simulink model "demodulate_16_bit1"  (R2021b)
settings: Solver=VariableStepAuto  StartTime=0.0  StopTime=100000/fs  RelTol=1e-3
PreLoadFcn:
  | clear all;
  | 
  | fs = 333e6
InitFcn:
  | fs = 333e6
libraries: hdlBasic x35, hdlsllib x3, dspsrcs4 x2, hdlUtilities x1, hdlDSPIP x1, simulink x1, vmcUtilities x1
settings Model: Creator=David Northcote  LastModifiedBy=clb20123
settings SolverCC: AlgebraicLoopSolver=TrustRegion
settings DataIOCC: ReturnWorkspaceOutputs=off
settings DebuggingCC: ArithmeticOperatorsInVariantConditions=warning
settings SFSimCC: SimUseLocalCustomCode=off  CustomCodeUndefinedFunction=UseInterfaceOnly
settings RTWCC: RTWUseLocalCustomCode=off  DLArmComputeVersion=20.02.1

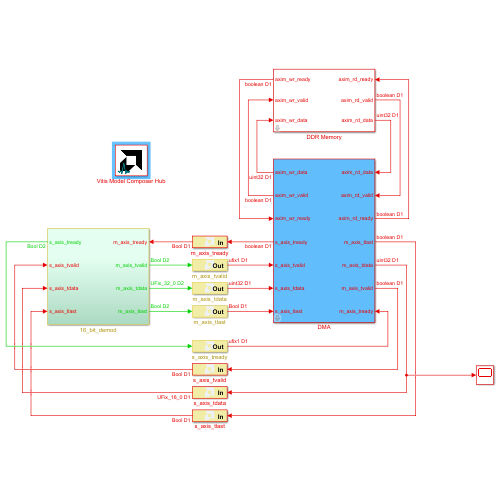
[thumbnail: Simulink's stored preview of the top-level diagram]
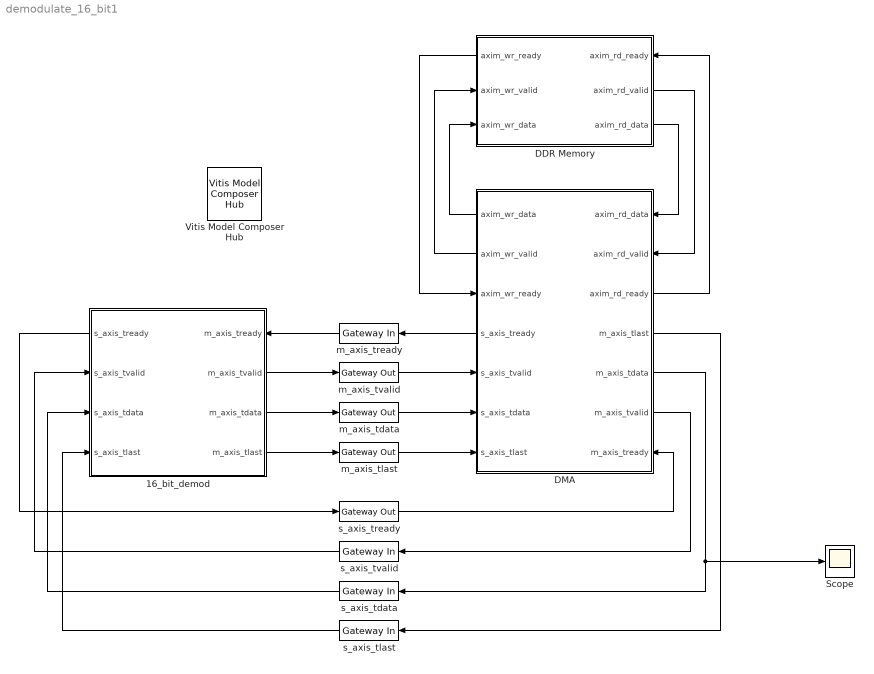
== system demodulate_16_bit1 ==
  16_bit_demod : Subsystem
      settings: PortSchema="{\"entries\":[{\"content\":{\"sides\":[{\"content\":{\"connectorIds\":[\"Out4\",\"In1\",\"In2\",\"In3\"]},\"type\":\"ConnectorPlacement.EquallySpacedRectSide\",\"uuid\":\"c102abcb-2e00-4fd7-85df-5b9b0b898bd0\"},{\"content\":{\"connectorIds\":[\"In4\",\"Out1\",\"Out2\",\"Out3\"],\"side\":\"RIGHT\"},\"type\":\"ConnectorPlacement.EquallySpacedRectSide\",\"uuid\":\"9e178eef-1e1d-41e3-971e-2eb7c6a5387e\"},{\"content\":{\"connectorIds\":[],\"side\":\"TOP\"},\"type\":\"ConnectorPlacement.EquallySpacedRectSide\",\"uuid\":\"12cf59e0-f07a-41d8-b174-5a1eb72b1624\"}]},\"type\":\"ConnectorPlacement.EquallySpacedConnector\",\"uuid\":\"cad21ed4-9065-49eb-a891-849a058d114a\"}],\"packageUris\":[\"http://schema.mathworks.com/mf0/Connector/19700101\"],\"version\":\"1.0\"}"
  DDR Memory : Subsystem  mask{bufferOut=[0 0 0 0 0 0 0 0 0 0 0], dtype=uint32, outVar='bufferIn'}
      mask prompts: bufferOut "Data to be sent:"; dtype "Data type:"; outVar "Output variable name:"
      mask init:
      | dtypeStr = get_param(gcb, 'dtype');
      | outVarStr = get_param(gcb, 'outVar');
      | set_param([gcb, '/Buffer In/To Workspace'], 'VariableName', outVar)
      settings: PortSchema="{\"entries\":[{\"content\":{\"sides\":[{\"content\":{\"connectorIds\":[\"Out3\",\"In1\",\"In2\"]},\"type\":\"ConnectorPlacement.EquallySpacedRectSide\",\"uuid\":\"10820561-fcd3-42da-ac38-14c6f993f770\"},{\"content\":{\"connectorIds\":[\"In3\",\"Out1\",\"Out2\"],\"side\":\"RIGHT\"},\"type\":\"ConnectorPlacement.EquallySpacedRectSide\",\"uuid\":\"072276f7-1cf8-495f-bb0a-1bca7e8326ea\"},{\"content\":{\"connectorIds\":[],\"side\":\"TOP\"},\"type\":\"ConnectorPlacement.EquallySpacedRectSide\",\"uuid\":\"f5b81d71-f8e7-451c-95ca-ef44dafc9f7a\"}]},\"type\":\"ConnectorPlacement.EquallySpacedConnector\",\"uuid\":\"59ea238c-ea64-4381-b9ec-a479227d5ff5\"}],\"packageUris\":[\"http://schema.mathworks.com/mf0/Connector/19700101\"],\"version\":\"1.0\"}"
      mask TypeOptions dtype: uint32 | int32
      mask DialogControl DescGroupVar Prompt: DDR Memory
      mask DialogControl DescTextVar Prompt: Block simulating a DDR memory controller.
      mask DialogControl ParameterGroupVar Prompt: MM2S
      mask DialogControl Container4 Prompt: S2MM
  DMA : Subsystem  mask{N=32}
      mask prompts: N "Length of data:"
      settings: PortSchema="{\"entries\":[{\"content\":{\"sides\":[{\"content\":{\"connectorIds\":[\"Out5\",\"Out6\",\"In1\",\"Out7\",\"In2\",\"In3\",\"In4\"]},\"type\":\"ConnectorPlacement.EquallySpacedRectSide\",\"uuid\":\"c102abcb-2e00-4fd7-85df-5b9b0b898bd0\"},{\"content\":{\"connectorIds\":[\"In5\",\"In6\",\"Out1\",\"Out2\",\"Out3\",\"Out4\",\"In7\"],\"side\":\"RIGHT\"},\"type\":\"ConnectorPlacement.EquallySpacedRectSide\",\"uuid\":\"9e178eef-1e1d-41e3-971e-2eb7c6a5387e\"},{\"content\":{\"connectorIds\":[],\"side\":\"TOP\"},\"type\":\"ConnectorPlacement.EquallySpacedRectSide\",\"uuid\":\"12cf59e0-f07a-41d8-b174-5a1eb72b1624\"},{\"content\":{\"connectorIds\":[],\"side\":\"BOTTOM\"},\"type\":\"ConnectorPlacement.EquallySpacedRectSide\",\"uuid\":\"a47cc6bb-72ec-4c9c-b625-c22428f6e2e0\"}]},\"type\":\"ConnectorPlacement.EquallySpacedConnector\",\"uuid\":\"cad21ed4-9065-49eb-a891-849a058d114a\"}],\"packageUris\":[\"http://schema.mathworks.com/mf0/Connector/19700101\"],\"version\":\"1.0\"}"
      mask DialogControl DescGroupVar Prompt: AXI DMA
      mask DialogControl DescTextVar Prompt: Block simulating an AXI DMA.
      mask DialogControl ParameterGroupVar Prompt: Main
  Scope : Scope
  Vitis Model Composer Hub : vmcUtilities/Vitis Model Composer Hub  Tag=genX  CodeGeneration=off  SubsystemName=16_bit_demod  DUTSubsystemName=16_bit_demod  CompilationType=HDLCompilation  ExportTypeV2=IP Catalog  TargetDirectory=./netlist\ip\16_bit_demod\src  exportDesign=on  analyzeDesign=off  validateDesignOnHw=off  ExportType=HDL  IpVendor=xilinx.com  IpLibrary=hls  IpVersion=1.0  IpHWLanguage=Verilog  AieCompilerOptions={}  AieSimulatorOptions={}  CreateTestbench=off  TestbenchStackSize=10  RunRtlSim=off  RunCSim=off  RunAieSim=off  AieSimTimeout=50000  RunAieSimProfiling=off  LaunchVitisAnalyzer=off  PlotOutput=off  RunX86Sim=off  X86SimTimeout=10  GenHwImage=off  GenLibadfXo=on  GenHwValidationCode=off  PlatformType=Not Specified  HwSystemType=Baremetal  HwValidationTarget=hw  ProjDevice=xczu43dr-fsve1156-2-e  ProjDevicePart=xczu43dr-fsve1156-2-e  SamplePeriod=-1  ClockFrequency=200  DataPathParallelism=1  xilinxfamily=zynquplusRFSOC  part=xczu43dr  speed=-2-e  package=fsve1156  directory=./netlist\ip\16_bit_demod\src  testbench=off  incr_netlist=off  synthesis_tool=Vivado  clock_wrapper=Clock Enables  dbl_ovrd=According to Block Masks  dcm_input_clock_period=10  sysclk_period=3.003  simulink_period=1/fs  eval_field=0  IPInfoJsonString="{\"HDLSubsystem\":{\"SubsystemName\":\"16_bit_demod\",\"IPName\":\"DUT\",\"IPLibrary\":\"VMC\",\"IPVendor\":\"User Company\",\"IPVersion\":\"1.0\",\"TargetDirectory\":\"./netlist\",\"SubsystemDir\":\"./netlist\\\\ip\\\\16_bit_demod\"},\"SubsystemTag\":\"HDLNode\"}"  LogFileName=''  NThreads=4
  m_axis_tdata : hdlBasic/Gateway Out  inherit_from_input=on  hdl_port=on  rows=1  columns=1  UseAsDAC=off  DACChannel='1'  interface=None  automatic_assignment=on  address_offset=hex2dec('00')  intf_name=''  intf_description=''  timing_constraint=None  locs_specified=off  LOCs={}  io_standard={}  XmcBlockStatus=1  maskContainerNames=group4  block_type=gatewayout  block_config=sysgen:gateway_out_config  block_width_w=590  block_height_w=620  block_width=620  block_height=750
  m_axis_tlast : hdlBasic/Gateway Out  inherit_from_input=on  hdl_port=on  rows=1  columns=1  UseAsDAC=off  DACChannel='1'  interface=None  automatic_assignment=on  address_offset=hex2dec('00')  intf_name=''  intf_description=''  timing_constraint=None  locs_specified=off  LOCs={}  io_standard={}  XmcBlockStatus=1  maskContainerNames=group4  block_type=gatewayout  block_config=sysgen:gateway_out_config  block_width_w=590  block_height_w=620  block_width=620  block_height=750
  m_axis_tready : hdlBasic/Gateway In  gui_display_data_type=Boolean  arith_type=Boolean  n_bits=16  bin_pt=14  preci_type=Single  exp_width=8  frac_width=24  rows=1  columns=1  quantization="Round  (unbiased: +/- Inf)"  overflow=Saturate  period=1/fs  UseAsADC=off  ADCChannel='1'  interface=None  automatic_assignment=on  address_offset=hex2dec('00')  intf_name=''  intf_description=''  default_value=0  timing_constraint=None  locs_specified=off  LOCs={}  io_standard={}  inherit_from_input=off  hdl_port=on  XmcBlockStatus=1  maskContainerNames=group4  block_type=gatewayin  block_config=sysgen:gateway_in_config  block_width_w=590  block_height_w=620  block_width=640  block_height=850
  m_axis_tvalid : hdlBasic/Gateway Out  inherit_from_input=on  hdl_port=on  rows=1  columns=1  UseAsDAC=off  DACChannel='1'  interface=None  automatic_assignment=on  address_offset=hex2dec('00')  intf_name=''  intf_description=''  timing_constraint=None  locs_specified=off  LOCs={}  io_standard={}  XmcBlockStatus=1  maskContainerNames=group4  block_type=gatewayout  block_config=sysgen:gateway_out_config  block_width_w=590  block_height_w=620  block_width=620  block_height=750
  s_axis_tdata : hdlBasic/Gateway In  gui_display_data_type=Fixed-point  arith_type=Unsigned  n_bits=16  bin_pt=0  preci_type=Single  exp_width=8  frac_width=24  rows=1  columns=1  quantization="Round  (unbiased: +/- Inf)"  overflow=Saturate  period=1/fs  UseAsADC=off  ADCChannel='1'  interface=None  automatic_assignment=on  address_offset=hex2dec('00')  intf_name=''  intf_description=''  default_value=0  timing_constraint=None  locs_specified=off  LOCs={}  io_standard={}  inherit_from_input=off  hdl_port=on  XmcBlockStatus=1  maskContainerNames=group4  block_type=gatewayin  block_config=sysgen:gateway_in_config  block_width_w=590  block_height_w=620  block_width=640  block_height=850
  s_axis_tlast : hdlBasic/Gateway In  gui_display_data_type=Boolean  arith_type=Boolean  n_bits=16  bin_pt=14  preci_type=Single  exp_width=8  frac_width=24  rows=1  columns=1  quantization="Round  (unbiased: +/- Inf)"  overflow=Saturate  period=1/fs  UseAsADC=off  ADCChannel='1'  interface=None  automatic_assignment=on  address_offset=hex2dec('00')  intf_name=''  intf_description=''  default_value=0  timing_constraint=None  locs_specified=off  LOCs={}  io_standard={}  inherit_from_input=off  hdl_port=on  XmcBlockStatus=1  maskContainerNames=group4  block_type=gatewayin  block_config=sysgen:gateway_in_config  block_width_w=590  block_height_w=620  block_width=640  block_height=850
  s_axis_tready : hdlBasic/Gateway Out  inherit_from_input=on  hdl_port=on  rows=1  columns=1  UseAsDAC=off  DACChannel='1'  interface=None  automatic_assignment=on  address_offset=hex2dec('00')  intf_name=''  intf_description=''  timing_constraint=None  locs_specified=off  LOCs={}  io_standard={}  XmcBlockStatus=1  maskContainerNames=group4  block_type=gatewayout  block_config=sysgen:gateway_out_config  block_width_w=590  block_height_w=620  block_width=620  block_height=750
  s_axis_tvalid : hdlBasic/Gateway In  gui_display_data_type=Boolean  arith_type=Boolean  n_bits=16  bin_pt=14  preci_type=Single  exp_width=8  frac_width=24  rows=1  columns=1  quantization="Round  (unbiased: +/- Inf)"  overflow=Saturate  period=1/fs  UseAsADC=off  ADCChannel='1'  interface=None  automatic_assignment=on  address_offset=hex2dec('00')  intf_name=''  intf_description=''  default_value=0  timing_constraint=None  locs_specified=off  LOCs={}  io_standard={}  inherit_from_input=off  hdl_port=on  XmcBlockStatus=1  maskContainerNames=group4  block_type=gatewayin  block_config=sysgen:gateway_in_config  block_width_w=590  block_height_w=620  block_width=640  block_height=850
  wires:
  s_axis_tvalid/1 -> 16_bit_demod/1(s_axis_tvalid)
  s_axis_tdata/1 -> 16_bit_demod/2(s_axis_tdata)
  s_axis_tlast/1 -> 16_bit_demod/3(s_axis_tlast)
  m_axis_tready/1 -> 16_bit_demod/4(m_axis_tready)
  16_bit_demod/4(s_axis_tready) -> s_axis_tready/1
  16_bit_demod/2(m_axis_tdata) -> m_axis_tdata/1
  16_bit_demod/1(m_axis_tvalid) -> m_axis_tvalid/1
  16_bit_demod/3(m_axis_tlast) -> m_axis_tlast/1
  s_axis_tready/1 -> DMA/7(m_axis_tready)
  DMA/4(m_axis_tvalid) -> s_axis_tvalid/1
  DMA/3(m_axis_tdata) -> Scope/1, s_axis_tdata/1
  DMA/2(m_axis_tlast) -> s_axis_tlast/1
  DMA/7(s_axis_tready) -> m_axis_tready/1
  m_axis_tvalid/1 -> DMA/2(s_axis_tvalid)
  m_axis_tdata/1 -> DMA/3(s_axis_tdata)
  m_axis_tlast/1 -> DMA/4(s_axis_tlast)
  DMA/1(axim_rd_ready) -> DDR Memory/3(axim_rd_ready)
  DDR Memory/1(axim_rd_valid) -> DMA/6(axim_rd_valid)
  DDR Memory/2(axim_rd_data) -> DMA/5(axim_rd_data)
  DDR Memory/3(axim_wr_ready) -> DMA/1(axim_wr_ready)
  DMA/6(axim_wr_valid) -> DDR Memory/1(axim_wr_valid)
  DMA/5(axim_wr_data) -> DDR Memory/2(axim_wr_data)

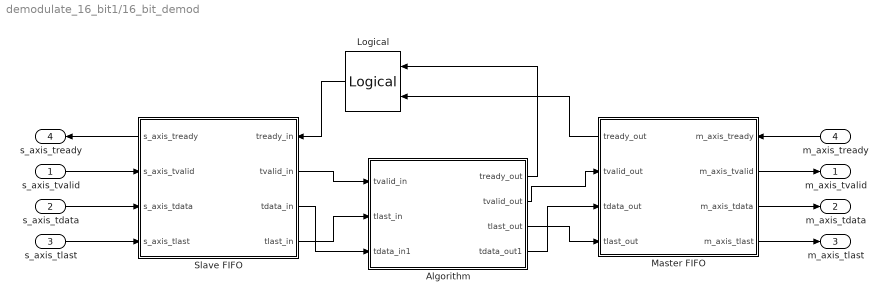
== system demodulate_16_bit1/16_bit_demod ==
  s_axis_tvalid : Inport
  s_axis_tdata : Inport  Port=2
  s_axis_tlast : Inport  Port=3
  m_axis_tready : Inport  Port=4
  Algorithm : Subsystem
  Logical : hdlBasic/Logical  logical_function=AND  inputs=2  en=off  latency=0  precision=Full  arith_type=Unsigned  n_bits=16  bin_pt=0  align_bp=on  overflow=[]  quantization=[]  XmcBlockStatus=1  maskContainerNames=tabcontainer1  block_type=logical  block_config=sysgen:Logical_config
  Master FIFO : Subsystem
      settings: PortSchema="{\"entries\":[{\"content\":{\"sides\":[{\"content\":{\"connectorIds\":[\"Out4\",\"In1\",\"In2\",\"In3\"]},\"type\":\"ConnectorPlacement.EquallySpacedRectSide\",\"uuid\":\"10820561-fcd3-42da-ac38-14c6f993f770\"},{\"content\":{\"connectorIds\":[\"In4\",\"Out1\",\"Out2\",\"Out3\"],\"side\":\"RIGHT\"},\"type\":\"ConnectorPlacement.EquallySpacedRectSide\",\"uuid\":\"072276f7-1cf8-495f-bb0a-1bca7e8326ea\"},{\"content\":{\"connectorIds\":[],\"side\":\"TOP\"},\"type\":\"ConnectorPlacement.EquallySpacedRectSide\",\"uuid\":\"f5b81d71-f8e7-451c-95ca-ef44dafc9f7a\"}]},\"type\":\"ConnectorPlacement.EquallySpacedConnector\",\"uuid\":\"59ea238c-ea64-4381-b9ec-a479227d5ff5\"}],\"packageUris\":[\"http://schema.mathworks.com/mf0/Connector/19700101\"],\"version\":\"1.0\"}"
  Slave FIFO : Subsystem
      settings: PortSchema="{\"entries\":[{\"content\":{\"sides\":[{\"content\":{\"connectorIds\":[\"Out4\",\"In1\",\"In2\",\"In3\"]},\"type\":\"ConnectorPlacement.EquallySpacedRectSide\",\"uuid\":\"10820561-fcd3-42da-ac38-14c6f993f770\"},{\"content\":{\"connectorIds\":[\"In4\",\"Out1\",\"Out2\",\"Out3\"],\"side\":\"RIGHT\"},\"type\":\"ConnectorPlacement.EquallySpacedRectSide\",\"uuid\":\"072276f7-1cf8-495f-bb0a-1bca7e8326ea\"},{\"content\":{\"connectorIds\":[],\"side\":\"TOP\"},\"type\":\"ConnectorPlacement.EquallySpacedRectSide\",\"uuid\":\"f5b81d71-f8e7-451c-95ca-ef44dafc9f7a\"}]},\"type\":\"ConnectorPlacement.EquallySpacedConnector\",\"uuid\":\"59ea238c-ea64-4381-b9ec-a479227d5ff5\"}],\"packageUris\":[\"http://schema.mathworks.com/mf0/Connector/19700101\"],\"version\":\"1.0\"}"
  m_axis_tvalid : Outport  VectorParamsAs1DForOutWhenUnconnected=off
  m_axis_tdata : Outport  Port=2  VectorParamsAs1DForOutWhenUnconnected=off
  m_axis_tlast : Outport  Port=3  VectorParamsAs1DForOutWhenUnconnected=off
  s_axis_tready : Outport  Port=4  VectorParamsAs1DForOutWhenUnconnected=off
  wires:
  Master FIFO/1(m_axis_tvalid) -> m_axis_tvalid/1
  Master FIFO/2(m_axis_tdata) -> m_axis_tdata/1
  Master FIFO/3(m_axis_tlast) -> m_axis_tlast/1
  Algorithm/2(tvalid_out) -> Master FIFO/1(tvalid_out)
  Algorithm/4(tdata_out1) -> Master FIFO/2(tdata_out)
  Algorithm/3(tlast_out) -> Master FIFO/3(tlast_out)
  s_axis_tvalid/1 -> Slave FIFO/1(s_axis_tvalid)
  s_axis_tdata/1 -> Slave FIFO/2(s_axis_tdata)
  s_axis_tlast/1 -> Slave FIFO/3(s_axis_tlast)
  Slave FIFO/1(tvalid_in) -> Algorithm/1(tvalid_in)
  Slave FIFO/3(tlast_in) -> Algorithm/2(tlast_in)
  Slave FIFO/4(s_axis_tready) -> s_axis_tready/1
  m_axis_tready/1 -> Master FIFO/4(m_axis_tready)
  Algorithm/1(tready_out) -> Logical/1
  Master FIFO/4(tready_out) -> Logical/2
  Logical/1 -> Slave FIFO/4(tready_in)
  Slave FIFO/2(tdata_in) -> Algorithm/3(tdata_in1)

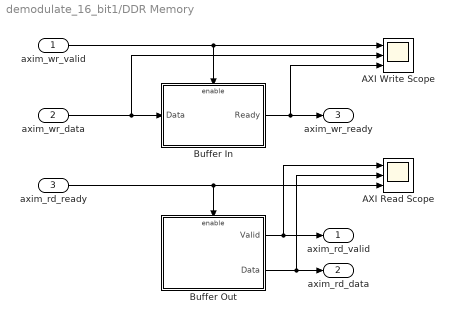
== system demodulate_16_bit1/DDR Memory ==
  axim_wr_valid : Inport
  axim_wr_data : Inport  Port=2
  axim_rd_ready : Inport  Port=3
  AXI Read Scope : Scope  NumInputPorts=3
  AXI Write Scope : Scope  NumInputPorts=3
  Buffer In : Subsystem
  Buffer Out : Subsystem
  axim_rd_valid : Outport
  axim_rd_data : Outport  Port=2
  axim_wr_ready : Outport  Port=3
  wires:
  Buffer Out/1(Valid) -> AXI Read Scope/1, axim_rd_valid/1
  Buffer Out/2(Data) -> AXI Read Scope/2, axim_rd_data/1
  axim_rd_ready/1 -> Buffer Out/Enable, AXI Read Scope/3
  axim_wr_data/1 -> AXI Write Scope/2, Buffer In/1(Data)
  Buffer In/1(Ready) -> AXI Write Scope/3, axim_wr_ready/1
  axim_wr_valid/1 -> Buffer In/Enable, AXI Write Scope/1

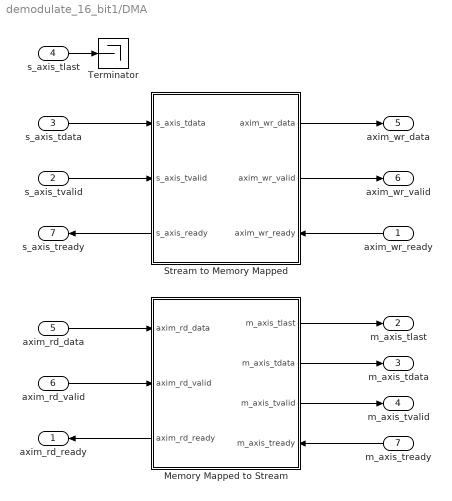
== system demodulate_16_bit1/DMA ==
  axim_wr_ready : Inport
  s_axis_tvalid : Inport  Port=2
  s_axis_tdata : Inport  Port=3
  s_axis_tlast : Inport  Port=4
  axim_rd_data : Inport  Port=5
  axim_rd_valid : Inport  Port=6
  m_axis_tready : Inport  Port=7
  Memory Mapped to Stream : Subsystem
      settings: PortSchema="{\"entries\":[{\"content\":{\"sides\":[{\"content\":{\"connectorIds\":[\"In1\",\"In2\",\"Out4\"]},\"type\":\"ConnectorPlacement.EquallySpacedRectSide\",\"uuid\":\"10820561-fcd3-42da-ac38-14c6f993f770\"},{\"content\":{\"connectorIds\":[\"Out1\",\"Out2\",\"Out3\",\"In3\"],\"side\":\"RIGHT\"},\"type\":\"ConnectorPlacement.EquallySpacedRectSide\",\"uuid\":\"072276f7-1cf8-495f-bb0a-1bca7e8326ea\"},{\"content\":{\"connectorIds\":[],\"side\":\"TOP\"},\"type\":\"ConnectorPlacement.EquallySpacedRectSide\",\"uuid\":\"f5b81d71-f8e7-451c-95ca-ef44dafc9f7a\"}]},\"type\":\"ConnectorPlacement.EquallySpacedConnector\",\"uuid\":\"59ea238c-ea64-4381-b9ec-a479227d5ff5\"}],\"packageUris\":[\"http://schema.mathworks.com/mf0/Connector/19700101\"],\"version\":\"1.0\"}"
  Stream to Memory Mapped : Subsystem
      settings: PortSchema="{\"entries\":[{\"content\":{\"sides\":[{\"content\":{\"connectorIds\":[\"In1\",\"In2\",\"Out3\"]},\"type\":\"ConnectorPlacement.EquallySpacedRectSide\",\"uuid\":\"10820561-fcd3-42da-ac38-14c6f993f770\"},{\"content\":{\"connectorIds\":[\"Out1\",\"Out2\",\"In3\"],\"side\":\"RIGHT\"},\"type\":\"ConnectorPlacement.EquallySpacedRectSide\",\"uuid\":\"072276f7-1cf8-495f-bb0a-1bca7e8326ea\"},{\"content\":{\"connectorIds\":[],\"side\":\"TOP\"},\"type\":\"ConnectorPlacement.EquallySpacedRectSide\",\"uuid\":\"f5b81d71-f8e7-451c-95ca-ef44dafc9f7a\"}]},\"type\":\"ConnectorPlacement.EquallySpacedConnector\",\"uuid\":\"59ea238c-ea64-4381-b9ec-a479227d5ff5\"}],\"packageUris\":[\"http://schema.mathworks.com/mf0/Connector/19700101\"],\"version\":\"1.0\"}"
  Terminator : Terminator
  axim_rd_ready : Outport
  m_axis_tlast : Outport  Port=2  VectorParamsAs1DForOutWhenUnconnected=off
  m_axis_tdata : Outport  Port=3  VectorParamsAs1DForOutWhenUnconnected=off
  m_axis_tvalid : Outport  Port=4  VectorParamsAs1DForOutWhenUnconnected=off
  axim_wr_data : Outport  Port=5
  axim_wr_valid : Outport  Port=6
  s_axis_tready : Outport  Port=7  VectorParamsAs1DForOutWhenUnconnected=off
  wires:
  m_axis_tready/1 -> Memory Mapped to Stream/3(m_axis_tready)
  Memory Mapped to Stream/1(m_axis_tlast) -> m_axis_tlast/1
  Memory Mapped to Stream/2(m_axis_tdata) -> m_axis_tdata/1
  Memory Mapped to Stream/3(m_axis_tvalid) -> m_axis_tvalid/1
  s_axis_tvalid/1 -> Stream to Memory Mapped/2(s_axis_tvalid)
  s_axis_tdata/1 -> Stream to Memory Mapped/1(s_axis_tdata)
  Stream to Memory Mapped/3(s_axis_ready) -> s_axis_tready/1
  s_axis_tlast/1 -> Terminator/1
  Stream to Memory Mapped/1(axim_wr_data) -> axim_wr_data/1
  Stream to Memory Mapped/2(axim_wr_valid) -> axim_wr_valid/1
  axim_wr_ready/1 -> Stream to Memory Mapped/3(axim_wr_ready)
  Memory Mapped to Stream/4(axim_rd_ready) -> axim_rd_ready/1
  axim_rd_data/1 -> Memory Mapped to Stream/1(axim_rd_data)
  axim_rd_valid/1 -> Memory Mapped to Stream/2(axim_rd_valid)

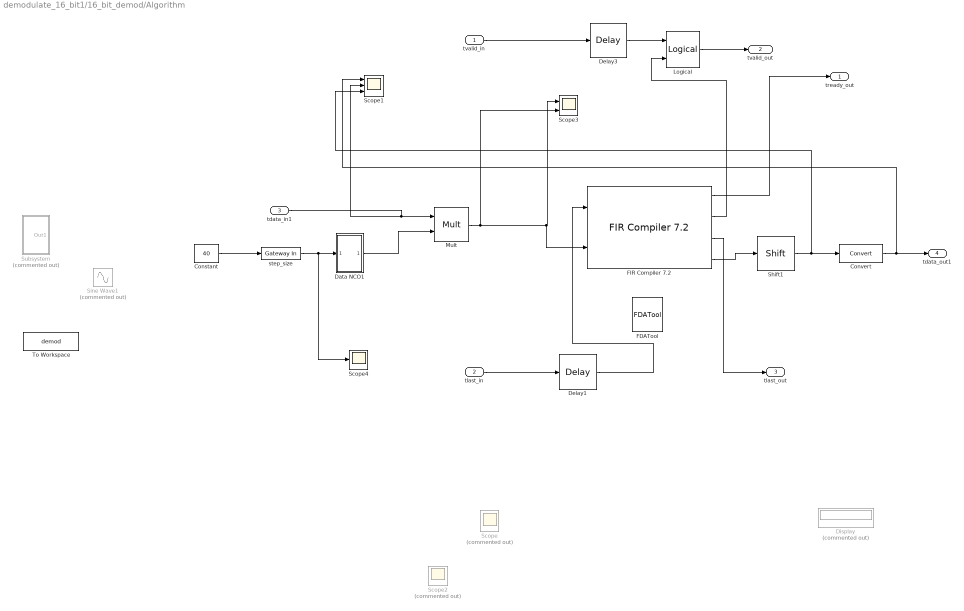
== system demodulate_16_bit1/16_bit_demod/Algorithm ==
  tvalid_in : Inport
  tlast_in : Inport  Port=2
  tdata_in1 : Inport  Port=3
  Constant : Constant  Value=40
  Convert : hdlBasic/Convert  gui_display_data_type=Fixed-point  arith_type=Unsigned  n_bits=32  bin_pt=0  float_type=Single  exp_bits=8  fraction_bits=24  quantization=Truncate  overflow=Wrap  en=off  latency=1  pipeline=off  XmcBlockStatus=1  maskContainerNames=group2  block_type=convert  block_config=sysgen:Convert_config  block_width=595  block_height=885
  Data NCO1 : Subsystem
  Delay1 : hdlBasic/Delay  rst=off  en=off  latency=9  reg_retiming=off  XmcBlockStatus=1  maskContainerNames=group1  block_type=delay  block_config=sysgen:Delay_config
  Delay3 : hdlBasic/Delay  rst=off  en=off  latency=9  reg_retiming=off  XmcBlockStatus=1  maskContainerNames=group1  block_type=delay  block_config=sysgen:Delay_config
  Display : Display  Commented=on
  FDATool : hdlUtilities/FDATool  block_type=fdatool
      settings: infoedit=FDATool
  FIR Compiler 7.2 : hdlDSPIP/FIR Compiler 7.2   coefficientvector=coeff  coefficient_sets=1  coefficient_reload=off  filter_type=Single_Rate  rate_change_type=Integer  interpolation_rate=1  decimation_rate=1  zero_pack_factor=1  channel_sequence=Basic  number_channels=1  pattern_list='P4-0,P4-1,P4-2,P4-3,P4-4'  number_paths=1  ratespecification=Maximum_Possible  sampleperiod=1  hardwareoversamplingrate=1  coefficient_sign=Signed  quantization=Normalize_to_Centre_Coefficient  coefficient_width=16  bestprecision=off  coefficient_fractional_bits=0  coefficient_structure=Inferred  output_rounding_mode=Full_Precision  output_width=31  filter_architecture=Systolic_Multiply_Accumulate  optimization_goal=Area  optimization_list='None'  data_buffer_type=Automatic  coefficient_buffer_type=Automatic  input_buffer_type=Automatic  output_buffer_type=Automatic  preference_for_other_storage=Automatic  multi_column_support=Automatic  columnconfig='101'  inter_column_pipe_length=4  data_has_tlast=Packet_Framing  m_data_has_tready=off  s_data_has_fifo=off  s_data_has_tuser=Not_Required  m_data_has_tuser=Not_Required  s_config_sync_mode=On_Vector  s_config_method=Single  num_reload_slots=1  has_aclken=off  has_aresetn=off  reset_data_vector=on  trim_axipin_name=on  simulation_type=hybrid_sim  simulation_model=sysgen:xfirv7_2_cmodel  data_path_portlist={ 's_axis_data_tdata', 'm_axis_data_tdata' }  passband_min=0.0  passband_max=0.5  stopband_min=0.5  stopband_max=1.0  filter_selection=1  gui_behaviour='Sysgen_GUI'  data_sign=Signed  data_width=16  data_fractional_bits=0  data_tuser_width=1  wrapper_available=true  ip_wrap_arbitrary_binary_point=true  ip_name=FIR Compiler  ip_version=7.2  dsptool_ready=true  ipcore_usecache=true  ipcore_useipmodelcache=true  port_translation_map={ 'aclken' => 'en', 'aresetn' => 'rst' }  run_core_at_system_period=true  ipcore_xco_need_fpga_part=true  ipcore_fpga_part=[]  XmcBlockStatus=1  maskContainerNames=tabcontainer1  block_type=fir_compiler_v7_2  block_config=sysgen:rodinimport_config  block_width=820  block_height=600
  Logical : hdlBasic/Logical  logical_function=AND  inputs=2  en=off  latency=0  precision=Full  arith_type=Unsigned  n_bits=16  bin_pt=0  align_bp=on  overflow=[]  quantization=[]  XmcBlockStatus=1  maskContainerNames=tabcontainer1  block_type=logical  block_config=sysgen:Logical_config
  Mult : hdlBasic/Mult  precision=Full  arith_type="Signed  (2's comp)"  n_bits=16  bin_pt=8  quantization=Truncate  overflow=Wrap  en=off  latency=3  use_behavioral_HDL=off  opt=Speed  use_embedded=on  optimum_pipeline=off  pipeline=on  use_rpm=on  placement_style=Triangular  XmcBlockStatus=1  maskContainerNames=group1  block_type=mult  block_config=sysgen:Mult_config  block_width=598  block_height=876
  Scope : Scope  Commented=on
  Scope1 : Scope  NumInputPorts=3
  Scope2 : Scope  Commented=on
  Scope3 : Scope  NumInputPorts=2
  Scope4 : Scope
  Shift1 : hdlBasic/Shift  shift_dir=Left  shift_bits=15  en=off  latency=1  precision=User Defined  arith_type="Signed  (2's comp)"  n_bits=47  bin_pt=0  quantization="Round  (unbiased: +/- Inf)"  overflow=Saturate  XmcBlockStatus=1  maskContainerNames=group2  block_type=shift  block_config=sysgen:Shift_config
  Sine Wave1 : Sin  Commented=on  Frequency=31415926.534298  SampleTime=0
  Subsystem : Subsystem  Commented=on
  To Workspace : ToWorkspace  VariableName=demod  SaveFormat=Timeseries  SampleTime=-1
  step_size : hdlBasic/Gateway In  gui_display_data_type=Fixed-point  arith_type=Signed (2's comp)  n_bits=16  bin_pt=8  preci_type=Single  exp_width=8  frac_width=24  rows=1  columns=1  quantization="Round  (unbiased: +/- Inf)"  overflow=Saturate  period=1/fs  UseAsADC=off  ADCChannel='1'  interface=None  automatic_assignment=on  address_offset=hex2dec('00')  intf_name=''  intf_description=''  default_value=0  timing_constraint=None  locs_specified=off  LOCs={}  io_standard={}  inherit_from_input=off  hdl_port=on  XmcBlockStatus=1  maskContainerNames=group4  block_type=gatewayin  block_config=sysgen:gateway_in_config  block_width_w=590  block_height_w=620  block_width=640  block_height=850
  tready_out : Outport
  tvalid_out : Outport  Port=2  VectorParamsAs1DForOutWhenUnconnected=off
  tlast_out : Outport  Port=3  VectorParamsAs1DForOutWhenUnconnected=off
  tdata_out1 : Outport  Port=4  VectorParamsAs1DForOutWhenUnconnected=off
  wires:
  tvalid_in/1 -> Delay3/1
  Delay1/1 -> FIR Compiler 7.2/1
  tlast_in/1 -> Delay1/1
  Delay3/1 -> Logical/1
  Logical/1 -> tvalid_out/1
  Shift1/1 -> Scope1/3, Convert/1
  step_size/1 -> Data NCO1/1(In1), Scope4/1
  Mult/1 -> FIR Compiler 7.2/2, Scope3/1, Scope3/2
  Constant/1 -> step_size/1
  Convert/1 -> tdata_out1/1, Scope1/1
  tdata_in1/1 -> Mult/1, Scope1/2
  Data NCO1/1(Out1) -> Mult/2
  FIR Compiler 7.2/2 -> Logical/2
  FIR Compiler 7.2/1 -> tready_out/1
  FIR Compiler 7.2/4 -> Shift1/1
  FIR Compiler 7.2/3 -> tlast_out/1

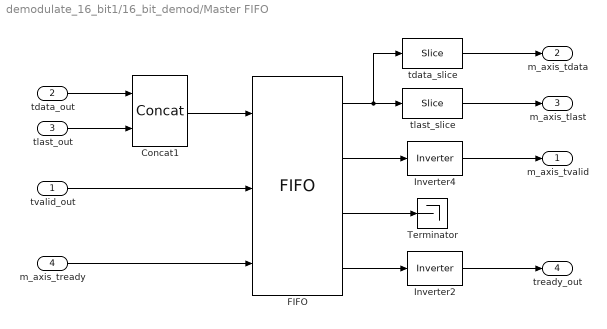
== system demodulate_16_bit1/16_bit_demod/Master FIFO ==
  tvalid_out : Inport
  tdata_out : Inport  Port=2
  tlast_out : Inport  Port=3
  m_axis_tready : Inport  Port=4
  Concat1 : hdlBasic/Concat  num_inputs=2  XmcBlockStatus=1  maskContainerNames=group1  block_type=concat  block_config=sysgen:Concat_config
  FIFO : hdlBasic/FIFO  mem_type=Block RAM  performance_options=First_Word_Fall_Through  embedded_registers=off  depth=1K  use_asym_data_widths=off  asym_read_width=32  percent_nbits=1  rst=off  rst_latency=2  en=off  use_dcount=off  use_percent_full_port=off  use_almost_empty=off  almost_empty_thresh=2  use_almost_full=on  use_rd_rst_busy=off  use_wr_rst_busy=off  almost_full_thresh=1000  almost_empty_offset=[]  almost_full_offset=[]  explicit_period=off  period=[]  store_only_valid=[]  init_zero=[]  simulation_type=fast_sim  XmcBlockStatus=1  maskContainerNames=tabcontainer1  block_type=fifo  block_config=sysgen:FIFO_config  block_width=538  block_height=997
      settings: infoedit=[]
  Inverter2 : hdlBasic/Inverter  en=off  latency=0  XmcBlockStatus=1  maskContainerNames=group2  block_type=inv  block_config=sysgen:Inverter_config
  Inverter4 : hdlBasic/Inverter  en=off  latency=0  XmcBlockStatus=1  maskContainerNames=group2  block_type=inv  block_config=sysgen:Inverter_config
  Terminator : Terminator
  tdata_slice : hdlBasic/Slice  nbits=1  boolean_output=off  mode=Two Bit Locations  bit1=0  base1=MSB of Input  bit0=1  base0=LSB of Input  XmcBlockStatus=1  maskContainerNames=group1  block_type=slice  block_config=sysgen:Slice_config
  tlast_slice : hdlBasic/Slice  nbits=1  boolean_output=on  mode=Two Bit Locations  bit1=0  base1=LSB of Input  bit0=0  base0=LSB of Input  XmcBlockStatus=1  maskContainerNames=group1  block_type=slice  block_config=sysgen:Slice_config
  m_axis_tvalid : Outport
  m_axis_tdata : Outport  Port=2
  m_axis_tlast : Outport  Port=3
  tready_out : Outport  Port=4
  wires:
  FIFO/4 -> Inverter2/1
  Inverter2/1 -> tready_out/1
  FIFO/2 -> Inverter4/1
  FIFO/1 -> tlast_slice/1, tdata_slice/1
  tlast_slice/1 -> m_axis_tlast/1
  tdata_slice/1 -> m_axis_tdata/1
  m_axis_tready/1 -> FIFO/3
  tvalid_out/1 -> FIFO/2
  Concat1/1 -> FIFO/1
  tdata_out/1 -> Concat1/1
  tlast_out/1 -> Concat1/2
  Inverter4/1 -> m_axis_tvalid/1
  FIFO/3 -> Terminator/1

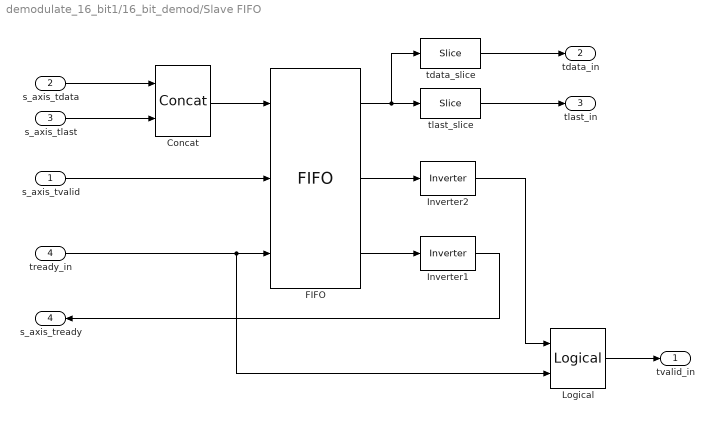
== system demodulate_16_bit1/16_bit_demod/Slave FIFO ==
  s_axis_tvalid : Inport
  s_axis_tdata : Inport  Port=2
  s_axis_tlast : Inport  Port=3
  tready_in : Inport  Port=4
  Concat : hdlBasic/Concat  num_inputs=2  XmcBlockStatus=1  maskContainerNames=group1  block_type=concat  block_config=sysgen:Concat_config
  FIFO : hdlBasic/FIFO  mem_type=Block RAM  performance_options=First_Word_Fall_Through  embedded_registers=off  depth=1K  use_asym_data_widths=off  asym_read_width=32  percent_nbits=1  rst=off  rst_latency=2  en=off  use_dcount=off  use_percent_full_port=off  use_almost_empty=off  almost_empty_thresh=2  use_almost_full=off  use_rd_rst_busy=off  use_wr_rst_busy=off  almost_full_thresh=14  almost_empty_offset=[]  almost_full_offset=[]  explicit_period=off  period=[]  store_only_valid=[]  init_zero=[]  simulation_type=fast_sim  XmcBlockStatus=1  maskContainerNames=tabcontainer1  block_type=fifo  block_config=sysgen:FIFO_config  block_width=538  block_height=997
      settings: infoedit=[]
  Inverter1 : hdlBasic/Inverter  en=off  latency=0  XmcBlockStatus=1  maskContainerNames=group2  block_type=inv  block_config=sysgen:Inverter_config
  Inverter2 : hdlBasic/Inverter  en=off  latency=0  XmcBlockStatus=1  maskContainerNames=group2  block_type=inv  block_config=sysgen:Inverter_config
  Logical : hdlBasic/Logical  logical_function=AND  inputs=2  en=off  latency=0  precision=Full  arith_type=Unsigned  n_bits=16  bin_pt=0  align_bp=on  overflow=[]  quantization=[]  XmcBlockStatus=1  maskContainerNames=tabcontainer1  block_type=logical  block_config=sysgen:Logical_config
  tdata_slice : hdlBasic/Slice  nbits=1  boolean_output=off  mode=Two Bit Locations  bit1=0  base1=MSB of Input  bit0=1  base0=LSB of Input  XmcBlockStatus=1  maskContainerNames=group1  block_type=slice  block_config=sysgen:Slice_config
  tlast_slice : hdlBasic/Slice  nbits=1  boolean_output=on  mode=Two Bit Locations  bit1=0  base1=LSB of Input  bit0=0  base0=LSB of Input  XmcBlockStatus=1  maskContainerNames=group1  block_type=slice  block_config=sysgen:Slice_config
  tvalid_in : Outport
  tdata_in : Outport  Port=2
  tlast_in : Outport  Port=3
  s_axis_tready : Outport  Port=4
  wires:
  FIFO/3 -> Inverter1/1
  s_axis_tvalid/1 -> FIFO/2
  tready_in/1 -> Logical/2, FIFO/3
  Concat/1 -> FIFO/1
  s_axis_tdata/1 -> Concat/1
  s_axis_tlast/1 -> Concat/2
  FIFO/1 -> tdata_slice/1, tlast_slice/1
  tlast_slice/1 -> tlast_in/1
  tdata_slice/1 -> tdata_in/1
  Inverter1/1 -> s_axis_tready/1
  FIFO/2 -> Inverter2/1
  Inverter2/1 -> Logical/1
  Logical/1 -> tvalid_in/1

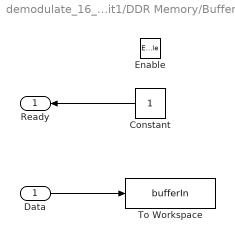
== system demodulate_16_bit1/DDR Memory/Buffer In ==
  Data : Inport
  Enable : EnablePort
  Constant : Constant  OutDataTypeStr=boolean  SampleTime=-1
  To Workspace : ToWorkspace  VariableName=bufferIn  SampleTime=-1
  Ready : Outport
  wires:
  Data/1 -> To Workspace/1
  Constant/1 -> Ready/1

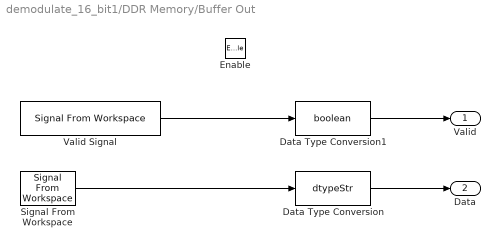
== system demodulate_16_bit1/DDR Memory/Buffer Out ==
  Enable : EnablePort
  Data Type Conversion : DataTypeConversion  OutDataTypeStr=dtypeStr
  Data Type Conversion1 : DataTypeConversion  OutDataTypeStr=boolean
  Signal From Workspace : dspsrcs4/Signal From Workspace  X=bufferOut  Ts=1/fs  nsamps=1  OutputAfterFinalValue=Setting to zero  ignoreOrWarnInputAndFrameLengths=off  OutputFrames=off
  Valid Signal : dspsrcs4/Signal From Workspace  X=ones(1, length(bufferOut))  Ts=1/fs  nsamps=1  OutputAfterFinalValue=Setting to zero  ignoreOrWarnInputAndFrameLengths=off  OutputFrames=off
  Valid : Outport
  Data : Outport  Port=2
  wires:
  Signal From Workspace/1 -> Data Type Conversion/1
  Data Type Conversion/1 -> Data/1
  Valid Signal/1 -> Data Type Conversion1/1
  Data Type Conversion1/1 -> Valid/1

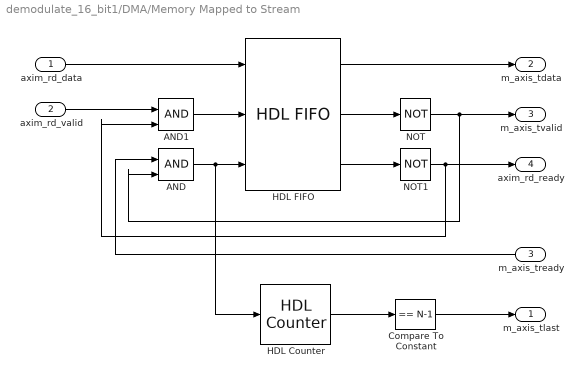
== system demodulate_16_bit1/DMA/Memory Mapped to Stream ==
  axim_rd_data : Inport
  axim_rd_valid : Inport  Port=2
  m_axis_tready : Inport  Port=3
  AND : Logic  IconShape=distinctive  AllPortsSameDT=off  OutDataTypeStr=boolean
  AND1 : Logic  IconShape=distinctive  AllPortsSameDT=off  OutDataTypeStr=boolean
  Compare To Constant : simulink/Logic and Bit Operations/Compare To Constant  relop===  const=N-1  OutDataTypeStr=boolean
  HDL Counter : hdlsllib/Sources/HDL Counter  CountType=Count limited  CountInit=0  CountStep=1  CountMax=N-1  CountFromType=Initial value  CountFrom=0  CountResetPort=off  CountLoadPort=off  CountEnbPort=on  CountDirPort=off  CountHitOutputPort=off  CountDataType=Unsigned  CountWordLen=ceil(log2(N))  CountFracLen=0  CountSampTime=1
  HDL FIFO : hdlsllib/HDL RAMs/HDL FIFO  fifo_size=16  mode=FWFT  ratio=1  push_msg=Warning  pop_msg=Warning  show_empty=on  show_full=on  show_num=off  LabelModeActiveChoice_Mode=FWFT
      settings: SourceProductBaseCode=SL
  NOT : Logic  Operator=NOT  IconShape=distinctive  AllPortsSameDT=off  OutDataTypeStr=boolean
  NOT1 : Logic  Operator=NOT  IconShape=distinctive  AllPortsSameDT=off  OutDataTypeStr=boolean
  m_axis_tlast : Outport  VectorParamsAs1DForOutWhenUnconnected=off
  m_axis_tdata : Outport  Port=2  VectorParamsAs1DForOutWhenUnconnected=off
  m_axis_tvalid : Outport  Port=3  VectorParamsAs1DForOutWhenUnconnected=off
  axim_rd_ready : Outport  Port=4  VectorParamsAs1DForOutWhenUnconnected=off
  wires:
  NOT/1 -> m_axis_tvalid/1, AND/2
  HDL Counter/1 -> Compare To Constant/1
  m_axis_tready/1 -> AND/1
  AND/1 -> HDL Counter/1, HDL FIFO/3
  Compare To Constant/1 -> m_axis_tlast/1
  HDL FIFO/2 -> NOT/1
  AND1/1 -> HDL FIFO/2
  HDL FIFO/1 -> m_axis_tdata/1
  HDL FIFO/3 -> NOT1/1
  NOT1/1 -> AND1/2, axim_rd_ready/1
  axim_rd_valid/1 -> AND1/1
  axim_rd_data/1 -> HDL FIFO/1

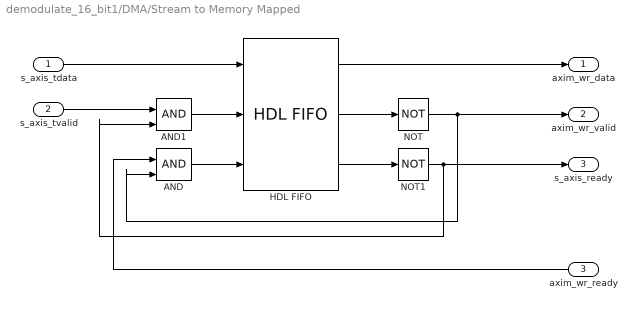
== system demodulate_16_bit1/DMA/Stream to Memory Mapped ==
  s_axis_tdata : Inport
  s_axis_tvalid : Inport  Port=2
  axim_wr_ready : Inport  Port=3
  AND : Logic  IconShape=distinctive  AllPortsSameDT=off  OutDataTypeStr=boolean
  AND1 : Logic  IconShape=distinctive  AllPortsSameDT=off  OutDataTypeStr=boolean
  HDL FIFO : hdlsllib/HDL RAMs/HDL FIFO  fifo_size=16  mode=FWFT  ratio=1  push_msg=Warning  pop_msg=Warning  show_empty=on  show_full=on  show_num=off  LabelModeActiveChoice_Mode=FWFT
      settings: SourceProductBaseCode=SL
  NOT : Logic  Operator=NOT  IconShape=distinctive  AllPortsSameDT=off  OutDataTypeStr=boolean
  NOT1 : Logic  Operator=NOT  IconShape=distinctive  AllPortsSameDT=off  OutDataTypeStr=boolean
  axim_wr_data : Outport  VectorParamsAs1DForOutWhenUnconnected=off
  axim_wr_valid : Outport  Port=2  VectorParamsAs1DForOutWhenUnconnected=off
  s_axis_ready : Outport  Port=3  VectorParamsAs1DForOutWhenUnconnected=off
  wires:
  s_axis_tvalid/1 -> AND1/1
  HDL FIFO/3 -> NOT1/1
  HDL FIFO/1 -> axim_wr_data/1
  AND1/1 -> HDL FIFO/2
  HDL FIFO/2 -> NOT/1
  AND/1 -> HDL FIFO/3
  axim_wr_ready/1 -> AND/1
  NOT/1 -> AND/2, axim_wr_valid/1
  s_axis_tdata/1 -> HDL FIFO/1
  NOT1/1 -> s_axis_ready/1, AND1/2

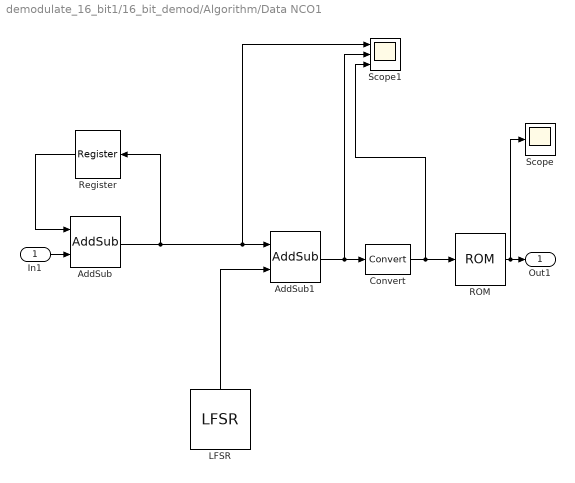
== system demodulate_16_bit1/16_bit_demod/Algorithm/Data NCO1 ==
  In1 : Inport
  AddSub : hdlBasic/AddSub  mode=Addition  use_carryin=off  use_carryout=off  en=off  latency=0  precision=User Defined  arith_type=Unsigned  n_bits=16  bin_pt=8  quantization="Round  (unbiased: +/- Inf)"  overflow=Wrap  use_behavioral_HDL=on  hw_selection=Fabric  pipelined=off  use_rpm=on  XmcBlockStatus=1  maskContainerNames=tabcontainer1  block_type=addsub  block_config=sysgen:Addsub_config
  AddSub1 : hdlBasic/AddSub  mode=Addition  use_carryin=off  use_carryout=off  en=off  latency=0  precision=User Defined  arith_type=Unsigned  n_bits=12  bin_pt=3  quantization=Truncate  overflow=Wrap  use_behavioral_HDL=on  hw_selection=Fabric  pipelined=off  use_rpm=on  XmcBlockStatus=1  maskContainerNames=tabcontainer1  block_type=addsub  block_config=sysgen:Addsub_config
  Convert : hdlBasic/Convert  gui_display_data_type=Fixed-point  arith_type=Unsigned  n_bits=8  bin_pt=0  float_type=Single  exp_bits=8  fraction_bits=24  quantization="Round  (unbiased: +/- Inf)"  overflow=Wrap  en=off  latency=1  pipeline=off  XmcBlockStatus=1  maskContainerNames=group2  block_type=convert  block_config=sysgen:Convert_config  block_width=595  block_height=885
  LFSR : hdlBasic/LFSR  lfsr_type=Galois  gate_type=XNOR  n_bits=16  maxpolynomial=on  polynomial='6805'  rst_value='03F'  rst=off  en=off  reloadable_seed=off  input_type=off  output_type=on  arith_type=Unsigned  bin_pt=16  explicit_period=off  period=1/fs  XmcBlockStatus=1  maskContainerNames=tabcontainer1  block_type=lfsr  block_config=sysgen:LFSR_config
  ROM : hdlBasic/ROM  depth=256  initVector=sin(pi*(0:255)/128)  distributed_mem=Block RAM  rst=off  init_reg=0  en=off  latency=1  gui_display_data_type=Fixed-point  arith_type="Signed  (2's comp)"  n_bits=16  bin_pt=15  preci_type=Single  exp_width=8  frac_width=24  optimize=Area  use_rpm=off  simulation_type=fast_sim  XmcBlockStatus=1  maskContainerNames=tabcontainer1  block_type=sprom  block_config=sysgen:SPROM_config
  Register : hdlBasic/Register  init=0  rst=off  en=off  XmcBlockStatus=1  maskContainerNames=tabcontainer1  block_type=register  block_config=sysgen:Register_config
  Scope : Scope
  Scope1 : Scope  NumInputPorts=3
  Out1 : Outport
  wires:
  In1/1 -> AddSub/2
  ROM/1 -> Scope/1, Out1/1
  Convert/1 -> Scope1/3, ROM/1
  LFSR/1 -> AddSub1/2
  AddSub/1 -> Scope1/1, AddSub1/1, Register/1
  Register/1 -> AddSub/1
  AddSub1/1 -> Scope1/2, Convert/1

== system demodulate_16_bit1/16_bit_demod/Algorithm/Subsystem ==
  Product : Product
  Sine Wave : Sin  Frequency=785398.1625000001  SampleTime=0
  Sine Wave1 : Sin  Frequency=31415926.534298  SampleTime=0
  Out1 : Outport
  wires:
  Product/1 -> Out1/1
  Sine Wave/1 -> Product/1
  Sine Wave1/1 -> Product/2
